simulink library "scndOrdTrnsThm_ul"  (R2018b)
settings: Solver=VariableStepAuto  StartTime=0.0  StopTime=10.0  RelTol=1e-3
libraries: vrlib x4
settings Model: Creator=mcobb  LastModifiedBy=mcobb

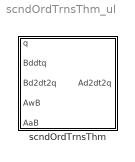
== system scndOrdTrnsThm_ul ==
  scndOrdTrnsThm : Subsystem

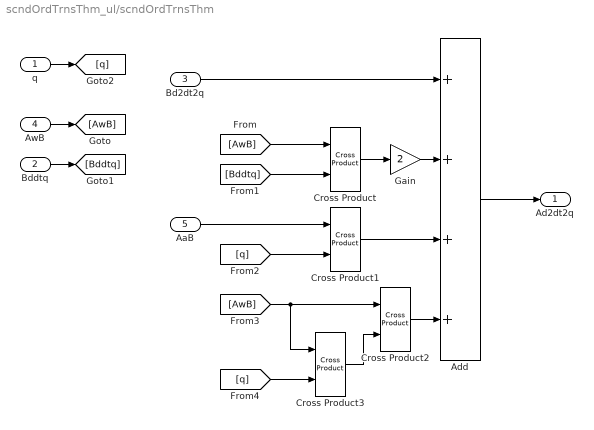
== system scndOrdTrnsThm_ul/scndOrdTrnsThm ==
  q : Inport  PortDimensions=3
  Bddtq : Inport  Port=2  PortDimensions=3
  Bd2dt2q : Inport  Port=3  PortDimensions=3
  AwB : Inport  Port=4  PortDimensions=3
  AaB : Inport  Port=5  PortDimensions=3
  Add : Sum  Inputs=++++
  Cross Product{,1..3} (4 alike) : vrlib/Utilities/Cross Product
      settings: SourceProductBaseCode=VR
  Gain : Gain  Gain=2
  Ad2dt2q : Outport
  wires:
  Add/1 -> Ad2dt2q/1
  Bd2dt2q/1 -> Add/1
  Cross Product/1 -> Gain/1
  AwB/1 -> [AwB]
  [AwB] -> Cross Product/1
  Bddtq/1 -> [Bddtq]
  [Bddtq] -> Cross Product/2
  AaB/1 -> Cross Product1/1
  Cross Product1/1 -> Add/3
  q/1 -> [q]
  [q] -> Cross Product1/2
  Gain/1 -> Add/2
  Cross Product2/1 -> Add/4
  [AwB] -> Cross Product3/1, Cross Product2/1
  Cross Product3/1 -> Cross Product2/2
  [q] -> Cross Product3/2
